simulink model "CruiseControlLogic"  (R2025a)
settings: Solver=VariableStepAuto  StartTime=0.0  StopTime=10.0  RelTol=1e-3
settings Model: Creator=nikul  LastModifiedBy=nikul

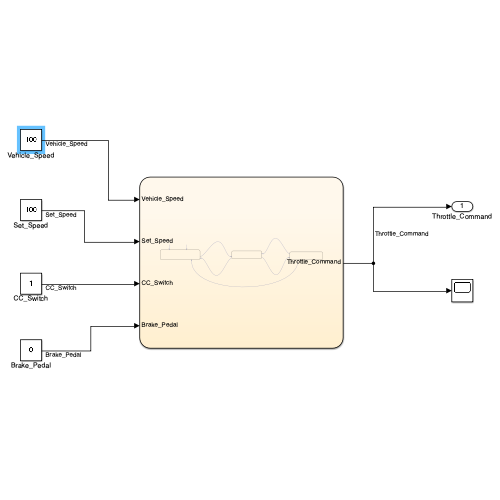
[thumbnail: Simulink's stored preview of the top-level diagram]
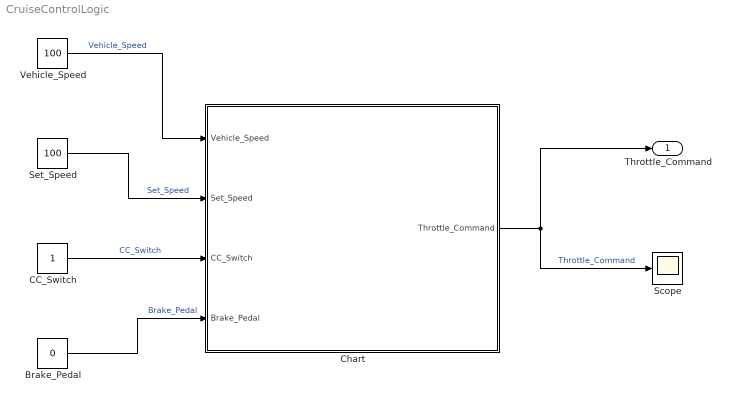
== system CruiseControlLogic ==
  Brake_Pedal : Constant  Value=0
  CC_Switch : Constant
  Chart : Stateflow chart  TreatAsAtomicUnit=on
  Scope : Scope
      settings: ActiveDisplayYMinimum=-0.12499999999999997  ActiveDisplayYMaximum=1.125
  Set_Speed : Constant  Value=100
  Vehicle_Speed : Constant  Value=100
  Throttle_Command : Outport
  wires:
  Vehicle_Speed/1 -> Chart/1(Vehicle_Speed)  "Vehicle_Speed"
  Set_Speed/1 -> Chart/2(Set_Speed)  "Set_Speed"
  CC_Switch/1 -> Chart/3(CC_Switch)  "CC_Switch"
  Brake_Pedal/1 -> Chart/4(Brake_Pedal)  "Brake_Pedal"
  Chart/1(Throttle_Command) -> Scope/1, Throttle_Command/1  "Throttle_Command"

== stateflow chart CruiseControlLogic/Chart ==
  state CC_OFF
    entry: Throttle_Command = 0;
  state CC_STANDBY
    entry: Throttle_Command = 0;
  state CC_ACTIVE
    entry: Throttle_Command = 1;
  CC_ACTIVE -> CC_STANDBY [order 1] : [Brake_Pedal == 1]
  CC_OFF -> CC_STANDBY : [CC_Switch == 1]
  (default) -> CC_OFF [order 1]
  (default) -> CC_OFF [order 2]
  CC_STANDBY -> CC_ACTIVE [order 2] : [Vehicle_Speed >= Set_Speed]
  CC_STANDBY -> CC_OFF [order 1] : [CC_Switch == 0]
  CC_ACTIVE -> CC_OFF [order 2] : [CC_Switch == 0]
  data: Vehicle_Speed input; Set_Speed input; CC_Switch input; Brake_Pedal input; Throttle_Command output
